simulink model "sampleModel1638"  (R2023a)
settings: Solver=VariableStepAuto  StartTime=0.0  StopTime=10.0  RelTol=1e-3
libraries: hdlsllib x4, simulink x3
settings Model: Creator=user1  LastModifiedBy=user1

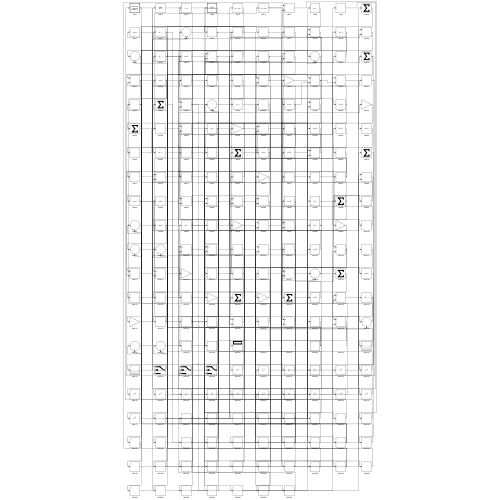
[thumbnail: Simulink's stored preview of the top-level diagram]
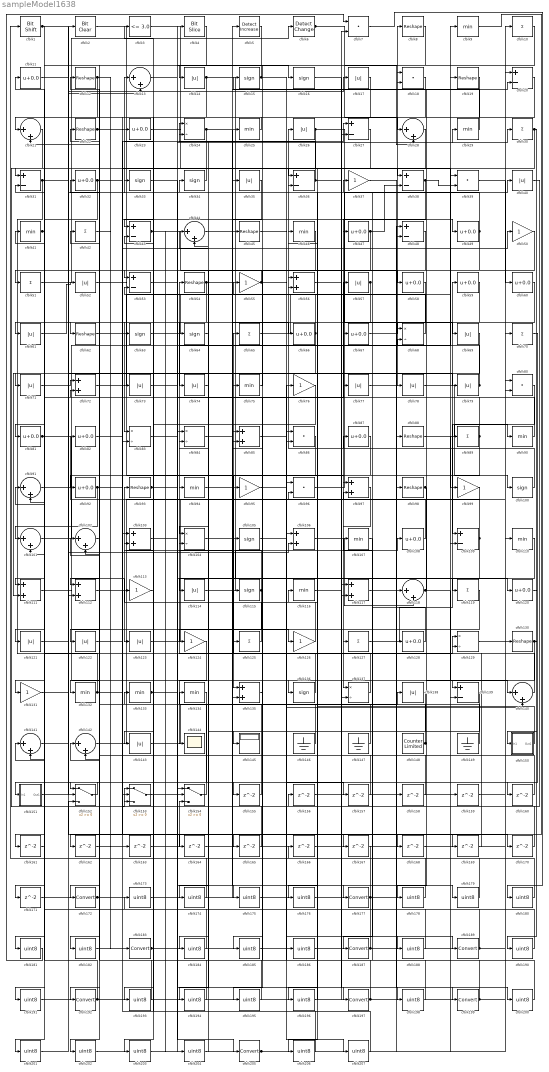
== system sampleModel1638 ==
  cfblk1 : hdlsllib/Logic and Bit Operations/Bit Shift  mode=Shift Left Logical  N=0
  cfblk{10,30,42,51,65,70,89,119,125,127} (10 alike) : Sum  Inputs=+
  cfblk{15..16,33..34,63..64,100,105,115,136} (10 alike) : Signum
  cfblk{13,21,28,44,91,101..102,118,140..142} (11 alike) : Sum  Inputs=|++
  cfblk{56,72,85,97,103,106,111..112,117,135} (10 alike) : Sum
  cfblk{24,68,83..84,104,129,137} (7 alike) : Product  Inputs=*/  RndMeth=Zero  SaturateOnIntegerOverflow=on
  cfblk{9,25,29,41,46,75,90,94,107,110,116,132..134} (14 alike) : MinMax
  cfblk{11,23,32,47,49,58..60,66..67,81..82,87,92,108,120,128} (17 alike) : Bias  Bias=0.0  SaturateOnIntegerOverflow=off
  cfblk{20,27,31,36,38,43,48,53,109,139} (10 alike) : Sum  Inputs=+-
  cfblk{37,50,55,76,95,99,113,124,126,131} (10 alike) : Gain
  cfblk{14,17,26,35,40,52,57,61,69,71,73..74,77..79,114,121..123,138,143} (21 alike) : Abs  SaturateOnIntegerOverflow=off
  cfblk{8,12,19,22,45,54,62,88,93,98,130} (11 alike) : Reshape
  cfblk144 : Scope
  cfblk145 : Display
  cfblk146 : Ground
  cfblk147 : Ground
  cfblk148 : hdlsllib/Sources/Counter Limited  uplimit=7  tsamp=-1
  cfblk149 : Ground
  cfblk150 : Subsystem
      settings: LibrarySourceBlock=|
      | hdlsllib/Ports &
      | Subsystems/Subsystem
  cfblk151 : Subsystem
      settings: LibrarySourceBlock=|
      | hdlsllib/Ports &
      | Subsystems/Subsystem
  cfblk152 : Switch  SaturateOnIntegerOverflow=off  InputSameDT=off
  cfblk153 : Switch  SaturateOnIntegerOverflow=off  InputSameDT=off
  cfblk154 : Switch  SaturateOnIntegerOverflow=off  InputSameDT=off
  cfblk{155..171} (17 alike) : Delay  SampleTime=1
  cfblk{172,177,183,187,189,192,197,199,205} (9 alike) : DataTypeConversion  SaturateOnIntegerOverflow=off  RndMeth=Floor
  cfblk{173..176,178..182,184..186,188,190..191,193..196,198,200..204,206..207} (27 alike) : DataTypeConversion  OutDataTypeStr=uint8  SaturateOnIntegerOverflow=off  RndMeth=Floor
  cfblk{7,18,39,80,86,96} (6 alike) : DotProduct  OutDataTypeStr=Inherit: Inherit via internal rule
  cfblk2 : simulink/Logic and Bit Operations/Bit Clear  iBit=0
      settings: LibrarySourceBlock=|
      | hdlsllib/Logic and Bit
      | Operations/Bit Clear
  cfblk3 : hdlsllib/Logic and Bit Operations/Compare To Constant  relop=<=  const=3.0  OutDataTypeStr=boolean
  cfblk4 : hdlsllib/Logic and Bit Operations/Bit Slice  lidx=7  ridx=0
  cfblk5 : simulink/Logic and Bit Operations/Detect Increase  vinit=0.0  OutDataTypeStr=boolean
      settings: LibrarySourceBlock=|
      | hdlsllib/Logic and Bit
      | Operations/Detect
      | Increase
  cfblk6 : simulink/Logic and Bit Operations/Detect Change  vinit=0  OutDataTypeStr=boolean
      settings: LibrarySourceBlock=|
      | hdlsllib/Logic and Bit
      | Operations/Detect
      | Change
  wires:
  cfblk51/1 -> cfblk6/1
  cfblk14/1 -> cfblk120/1, cfblk193/1
  cfblk125/1 -> cfblk93/1
  cfblk31/1 -> cfblk129/1, cfblk170/1
  cfblk38/1 -> cfblk137/1, cfblk39/2
  cfblk136/1 -> cfblk54/1
  cfblk29/1 -> cfblk62/1
  cfblk140/1 -> cfblk65/1
  cfblk106/1 -> cfblk118/2
  cfblk114/1 -> cfblk108/1
  cfblk61/1 -> cfblk52/1
  cfblk52/1 -> cfblk135/1
  cfblk100/1 -> cfblk26/1
  cfblk70/1 -> cfblk152/1
  cfblk42/1 -> cfblk183/1
  cfblk142/1 -> cfblk105/1
  cfblk78/1 -> cfblk100/1
  cfblk127/1 -> cfblk59/1
  cfblk5/1 -> cfblk172/1
  cfblk84/1 -> cfblk177/1
  cfblk96/1 -> cfblk40/1
  cfblk2/1 -> cfblk97/1
  cfblk115/1 -> cfblk94/1, cfblk124/1
  cfblk66/1 -> cfblk3/1, cfblk111/2, cfblk164/1
  cfblk143/1 -> cfblk138/1
  cfblk67/1 -> cfblk8/1
  cfblk49/1 -> cfblk13/1, cfblk73/1
  cfblk97/1 -> cfblk127/1
  cfblk101/1 -> cfblk9/1
  cfblk37/1 -> cfblk199/1
  cfblk141/1 -> cfblk106/2
  cfblk137/1 -> cfblk125/1
  cfblk72/1 -> cfblk56/1
  cfblk55/1 -> cfblk51/1, cfblk207/1
  cfblk54/1 -> cfblk66/1, cfblk181/1
  cfblk80/1 -> cfblk109/1
  cfblk112/1 -> cfblk70/1
  cfblk126/1 -> cfblk34/1
  cfblk81/1 -> cfblk126/1, cfblk13/2
  cfblk129/1 -> cfblk130/1
  cfblk111/1 -> cfblk139/1
  cfblk21/1 -> cfblk153/1
  cfblk68/1 -> cfblk15/1
  cfblk57/1 -> cfblk83/1, cfblk131/1
  cfblk95/1 -> cfblk197/1
  cfblk102/1 -> cfblk192/1
  cfblk122/1 -> cfblk63/1
  cfblk123/1 -> cfblk76/1
  cfblk135/1 -> cfblk85/1
  cfblk89/1 -> cfblk41/1, cfblk92/1
  cfblk20/1 -> cfblk71/1
  cfblk107/1 -> cfblk187/1
  cfblk151/1(Out1) -> cfblk33/1
  cfblk146/1 -> cfblk75/1
  cfblk58/1 -> cfblk74/1
  cfblk104/1 -> cfblk25/1
  cfblk152/1 -> cfblk151/1(In1)
  cfblk150/1(Out1) -> cfblk116/1
  cfblk153/1 -> cfblk30/1
  cfblk3/1 -> cfblk86/2
  cfblk131/1 -> cfblk2/1
  cfblk27/1 -> cfblk43/1
  cfblk12/1 -> cfblk101/1, cfblk163/1
  cfblk65/1 -> cfblk19/1
  cfblk59/1 -> cfblk78/1
  cfblk117/1 -> cfblk189/1
  cfblk88/1 -> cfblk90/1
  cfblk94/1 -> cfblk45/1
  cfblk18/1 -> cfblk83/2
  cfblk93/1 -> cfblk29/1, cfblk77/1
  cfblk74/1 -> cfblk104/1
  cfblk43/1 -> cfblk158/1, cfblk204/1
  cfblk119/1 -> cfblk145/1
  cfblk26/1 -> cfblk69/1, cfblk182/1
  cfblk11/1 -> cfblk152/2
  cfblk10/1 -> cfblk121/1
  cfblk53/1 -> cfblk135/2
  cfblk28/1 -> cfblk112/1
  cfblk109/1 -> cfblk24/1, cfblk194/1, cfblk196/1
  cfblk75/1 -> cfblk55/1
  cfblk108/1 -> cfblk82/1
  cfblk76/1 -> cfblk143/1
  cfblk71/1 -> cfblk72/1
  cfblk69/1 -> cfblk115/1
  cfblk34/1 -> cfblk31/1
  cfblk99/1 -> cfblk96/2
  cfblk36/1 -> cfblk137/2, cfblk24/2
  cfblk23/1 -> cfblk36/1
  cfblk91/1 -> cfblk123/1
  cfblk33/1 -> cfblk119/1
  cfblk148/1 -> cfblk22/1, cfblk67/1
  cfblk17/1 -> cfblk132/1
  cfblk41/1 -> cfblk81/1, cfblk101/2
  cfblk90/1 -> cfblk57/1
  cfblk8/1 -> cfblk112/2
  cfblk154/1 -> cfblk133/1
  cfblk1/1 -> cfblk79/1, cfblk191/1
  cfblk44/1 -> cfblk20/2
  cfblk6/1 -> cfblk28/1, cfblk28/2
  cfblk50/1 -> cfblk53/1
  cfblk35/1 -> cfblk85/2
  cfblk25/1 -> cfblk21/1
  cfblk132/1 -> cfblk136/1, cfblk11/1
  cfblk130/1 -> cfblk150/1(In1), cfblk168/1
  cfblk103/1 -> cfblk205/1
  cfblk39/1 -> cfblk60/1
  cfblk63/1 -> cfblk39/1
  cfblk62/1 -> cfblk27/1
  cfblk56/1 -> cfblk58/1
  cfblk77/1 -> cfblk88/1
  cfblk47/1 -> cfblk122/1, cfblk38/2
  cfblk147/1 -> cfblk43/2
  cfblk124/1 -> cfblk144/1
  cfblk64/1 -> cfblk114/1
  cfblk149/1 -> cfblk32/1
  cfblk60/1 -> cfblk142/2
  cfblk98/1 -> cfblk18/1, cfblk178/1
  cfblk118/1 -> cfblk140/1, cfblk18/2
  cfblk22/1 -> cfblk99/1, cfblk38/1
  cfblk128/1 -> cfblk87/1
  cfblk133/1 -> cfblk68/2, cfblk179/1
  cfblk30/1 -> cfblk190/1, cfblk206/1
  cfblk15/1 -> cfblk14/1, cfblk140/2
  cfblk24/1 -> cfblk49/1, cfblk202/1
  cfblk121/1 -> cfblk17/1
  cfblk79/1 -> cfblk44/2, cfblk36/2
  cfblk13/1 -> cfblk16/1
  cfblk92/1 -> cfblk50/1, cfblk171/1
  cfblk32/1 -> cfblk47/1, cfblk61/1, cfblk111/1
  cfblk113/1 -> cfblk23/1
  cfblk87/1 -> cfblk155/1
  cfblk155/1 -> cfblk72/2
  cfblk40/1 -> cfblk156/1
  cfblk156/1 -> cfblk109/2
  cfblk85/1 -> cfblk157/1
  cfblk157/1 -> cfblk104/2
  cfblk158/1 -> cfblk44/1
  cfblk159/1 -> cfblk80/1
  cfblk120/1 -> cfblk160/1
  cfblk160/1 -> cfblk21/2
  cfblk19/1 -> cfblk161/1
  cfblk161/1 -> cfblk141/2
  cfblk9/1 -> cfblk162/1
  cfblk162/1 -> cfblk118/1
  cfblk163/1 -> cfblk154/3
  cfblk164/1 -> cfblk20/1
  cfblk86/1 -> cfblk165/1
  cfblk165/1 -> cfblk153/2
  cfblk166/1 -> cfblk56/2
  cfblk82/1 -> cfblk167/1
  cfblk167/1 -> cfblk1/1
  cfblk168/1 -> cfblk139/2
  cfblk116/1 -> cfblk169/1
  cfblk169/1 -> cfblk129/2
  cfblk170/1 -> cfblk153/3
  cfblk171/1 -> cfblk68/1
  cfblk172/1 -> cfblk27/2, cfblk35/1
  cfblk173/1 -> cfblk5/1
  cfblk48/1 -> cfblk174/1
  cfblk174/1 -> cfblk12/1
  cfblk83/1 -> cfblk175/1
  cfblk175/1 -> cfblk48/1
  cfblk138/1 -> cfblk176/1
  cfblk176/1 -> cfblk48/2
  cfblk177/1 -> cfblk173/1, cfblk96/1
  cfblk178/1 -> cfblk84/1
  cfblk179/1 -> cfblk84/2
  cfblk7/1 -> cfblk180/1
  cfblk180/1 -> cfblk141/1
  cfblk181/1 -> cfblk7/1
  cfblk182/1 -> cfblk7/2
  cfblk183/1 -> cfblk113/1, cfblk106/1
  cfblk139/1 -> cfblk184/1
  cfblk184/1 -> cfblk42/1
  cfblk110/1 -> cfblk185/1
  cfblk185/1 -> cfblk98/1
  cfblk45/1 -> cfblk186/1
  cfblk186/1 -> cfblk110/1
  cfblk187/1 -> cfblk166/1, cfblk53/2, cfblk97/2
  cfblk105/1 -> cfblk188/1
  cfblk188/1 -> cfblk107/1
  cfblk189/1 -> cfblk91/2, cfblk31/2, cfblk154/2
  cfblk190/1 -> cfblk117/1
  cfblk191/1 -> cfblk117/2
  cfblk192/1 -> cfblk91/1, cfblk10/1
  cfblk193/1 -> cfblk102/1
  cfblk194/1 -> cfblk102/2
  cfblk46/1 -> cfblk195/1
  cfblk195/1 -> cfblk154/1
  cfblk196/1 -> cfblk46/1
  cfblk197/1 -> cfblk89/1, cfblk86/1
  cfblk73/1 -> cfblk198/1
  cfblk198/1 -> cfblk95/1
  cfblk199/1 -> cfblk64/1, cfblk142/1
  cfblk16/1 -> cfblk200/1
  cfblk200/1 -> cfblk37/1
  cfblk4/1 -> cfblk201/1
  cfblk201/1 -> cfblk152/3
  cfblk202/1 -> cfblk4/1
  cfblk134/1 -> cfblk203/1
  cfblk203/1 -> cfblk159/1
  cfblk204/1 -> cfblk134/1
  cfblk205/1 -> cfblk80/2, cfblk128/1
  cfblk206/1 -> cfblk103/1
  cfblk207/1 -> cfblk103/2

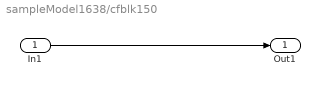
== system sampleModel1638/cfblk150 ==
  In1 : Inport
  Out1 : Outport
  wires:
  In1/1 -> Out1/1

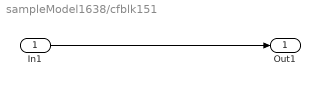
== system sampleModel1638/cfblk151 ==
  In1 : Inport
  Out1 : Outport
  wires:
  In1/1 -> Out1/1
